simulink model "PMSMWithThermal"  (R2024b)
settings: Solver=VariableStepAuto  StartTime=0.0  StopTime=5  RelTol=1e-3  AbsTol=1e-3
PreLoadFcn:
  | PMSMWithThermalParameters;
values from neighbouring files (symbols this model uses):
  B = 0    [param.mat]
  dt = 0.5e-4    (= 5e-05)    [PMSMWithThermalParameters.m]    (also in param.mat)
  dt_speed_control = 0.001    [PMSMWithThermalParameters.m]    (also in param.mat)
  ESO_w0 = 0    [param.mat]
  J = 0.02    [param.mat]
  max_power = 50e3    (= 50000)    [PMSMWithThermalParameters.m]    (also in param.mat)
  max_torque = 220    [PMSMWithThermalParameters.m]    (also in param.mat)
  N = 6    [PMSMWithThermalParameters.m]    (also in param.mat)
  Rs = 0.013    [PMSMWithThermalParameters.m]    (also in param.mat = 1.3)
undefined symbols (not defined in the file or in its folder): DiscIntNeverNeededParam
libraries: fl_lib x124, nesl_utility x33, fl_ps_legacy_lib x3, ee_lib x1, simulink x1
(part 1 of 2)
CloseFcn:
  | try,close(h1_PMSMWithThermal),end
  | clear h1_PMSMWithThermal
  | try,close(h2_PMSMWithThermal),end
  | clear h2_PMSMWithThermal
  | 
  | 
  | clear simlog_PMSMWithThermal
  | clear logsout_PMSMWithThermal
  | clear Lm Ls Ms N PM Rs dfluxdiMatrix dfluxdxMatrix dt dt_speed_control iVec_th max_power max_torque ni nx row row_PM row_RM tout w_max_power xVecRad xVec_th
Description:
  | PMSM with Thermal Model
settings Model: Creator=The MathWorks, Inc.  LastModifiedBy=Yusuke Seki
settings SolverCC: AutoScaleAbsTol=off  AlgebraicLoopSolver=TrustRegion  MaxZcPerStep=1
settings DataIOCC: MaxDataPoints=210000  SaveFormat=Array  SignalLoggingName=logsout_PMSMWithThermal
settings OptimizationCC: BlockReduction=off  BooleanDataType=off  ReuseModelBlockBuffer=off  LifeSpan=inf
settings DebuggingCC: SaveWithParameterizedLinksMsg=none  SignalResolutionControl=TryResolveAllWithWarning  UnconnectedInputMsg=warning  UnconnectedOutputMsg=warning  UnconnectedLineMsg=warning  AllowSymbolicDim=off  SFUnexpectedBacktrackingDiag=warning  SFNoUnconditionalDefaultTransitionDiag=warning  SFExecutionAtInitializationDiag=none  ArithmeticOperatorsInVariantConditions=warning
settings HardwareCC: ProdBitPerPointer=32  ProdBitPerSizeT=32  ProdBitPerPtrDiffT=32  ProdLargestAtomicFloat=None  ProdIntDivRoundTo=Undefined  ProdEndianess=Unspecified  ProdWordSize=32  ProdHWDeviceType=32-bit Generic  TargetUnknown=on
settings ModelReferenceCC: EnableRefExpFcnMdlSchedulingChecks=on  PropagateSignalLabelsOutOfModel=off
settings SFSimCC: SimUseLocalCustomCode=off  CustomCodeUndefinedFunction=UseInterfaceOnly
settings RTWCC: RTWUseLocalCustomCode=off  GPUComputeCapability=3.5  DLArmComputeVersion=19.05
settings CodeAppCC: StateflowObjectComments=on
settings GRTTargetCC: TargetLangStandard=C89/C90 (ANSI)
settings ConfigComp: CovMetricSettings=dw  CovSaveCumulativeToWorkspaceVar=on  CovSaveSingleToWorkspaceVar=on  CovExternalEMLEnable=off  CovSFcnEnable=off
settings SimscapeCC: SimscapeLogType=all  SimscapeLogSimulationStatistics=on  SimscapeLogName=simlog_PMSMWithThermal  SimscapeLogDecimation=10  SimscapeLogDataHistory=210000

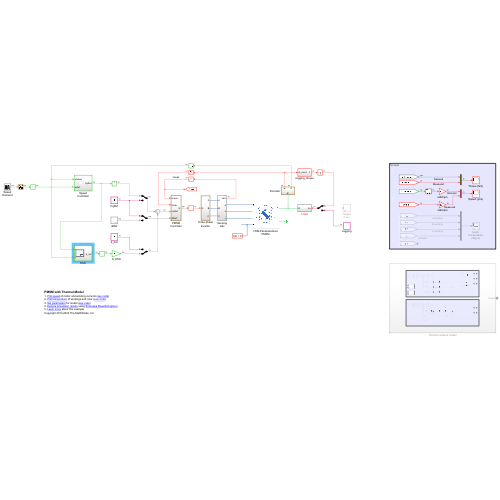
[thumbnail: Simulink's stored preview of the top-level diagram]
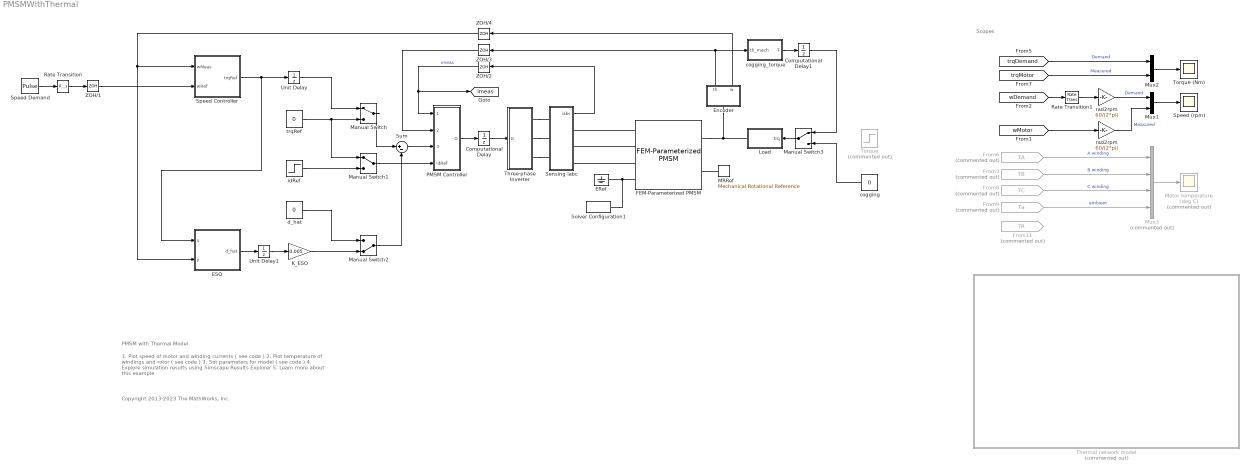
== system PMSMWithThermal ==
  note: Scopes
  note: PMSM with Thermal Model
  note: 1. Plot speed of motor and winding currents ( see code )
      | 2. Plot temperature of windings and rotor ( see code )
      | 3. Set parameters for model ( see code )
      | 4. Explore simulation results using Simscape Results Explorer
      | 5. Learn more about this example
  note: Copyright 2013-2023 The MathWorks, Inc.
  " rad2rpm " : Gain  Gain=60/(2*pi)
  Computational Delay : UnitDelay  SampleTime=dt  HasFrameUpgradeWarning=on
  Computational Delay1 : UnitDelay  SampleTime=dt  HasFrameUpgradeWarning=on
  ERef : fl_lib/Electrical/Electrical Elements/Electrical Reference
  ESO : Subsystem  TreatAsAtomicUnit=on  SystemSampleTime=dt_speed_control
  Encoder : Subsystem
  FEM-Parameterized PMSM : ee_lib/Electromechanical/Permanent Magnet/FEM-Parameterized PMSM  parameterization=ee.enum.fem_motor.parameterization.sinusoidalBackEMF  winding_type=ee.enum.statorconnection.wye  iVec=iVec_th A  xVec=xVec_th deg  dfluxdiMatrix=dfluxdiMatrix Wb/A  dfluxdxMatrix=dfluxdxMatrix Wb/rad  calculate_torque_matrix=1  TorqueMatrix=[0, 0.3, - 0.3, 0; 0, 0, 0, 0; 0, - 0.3, 0.3, 0] N*m  idVec1=[-200.0, 0.0, 200.0] A  iqVec1=[-200.0, 0.0, 200.0] A  LdMatrix=0.0002 * ones(3, 3) H  LqMatrix=0.0002 * ones(3, 3) H  PmMatrix=0.1 * ones(3, 3) Wb  interp_method=1  N=N  Rs=Rs Ohm  Ms=Ms H  L0=0.00016 H  loss_param=ee.enum.fem_motor.ironLosses.none  losses_oc=[0.0, 0.0, 0.0] W  losses_sc=[0.0, 0.0, 0.0] W  f_losses=60 Hz  Isc_losses=95 A  Inertia=J kg*m^2  lam=B N*m/(rad/s)  i_d_specify=off  i_d_priority=None  i_d=0 A  i_d_nominal_specify=off  i_d_nominal_value=1  i_d_nominal_unit=A  i_q_specify=off  i_q_priority=None  i_q=0 A  i_q_nominal_specify=off  i_q_nominal_value=1  i_q_nominal_unit=A  torque_specify=off  torque_priority=None  torque=0 N*m  torque_nominal_specify=off  torque_nominal_value=1  torque_nominal_unit=N*m  angular_velocity_specify=on  angular_velocity_priority=High  angular_velocity=0 rpm  angular_velocity_nominal_specify=off  angular_velocity_nominal_value=1  angular_velocity_nominal_unit=rpm  angular_position_specify=on  angular_position_priority=High  angular_position=0 deg  angular_position_nominal_specify=off  angular_position_nominal_value=1  angular_position_nominal_unit=deg  alpha=3.93e-3 1/K  alpha_flux=-0.001 1/K  Tmeas=298.15 K  stator_thermal_mass=2 J/K  stator_initial_temperatures=[298.15, 298.15, 298.15] K  rotor_thermal_mass=20 J/K  rotor_initial_temperature=298.15 K  Rm_percent_rotor=90  Rd_percent_rotor=30  idVec=[-200, 0, 200] A  iqVec=[-200, 0, 200] A  dfluxAdiaMatrix3D=zeros(3, 3, 4) Wb/A  dfluxAdibMatrix3D=zeros(3, 3, 4) Wb/A  dfluxAdicMatrix3D=zeros(3, 3, 4) Wb/A  dfluxAdxMatrix3D=zeros(3, 3, 4) Wb/rad  TorqueMatrix3D=zeros(3, 3, 4) N*m  iaVec=[-200, 0, 200] A  ibVec=[-200, 0, 200] A  icVec=[-200, 0, 200] A  dfluxAdiaMatrix=zeros(3, 3, 3, 4) Wb/A  dfluxAdibMatrix=zeros(3, 3, 3, 4) Wb/A  dfluxAdicMatrix=zeros(3, 3, 3, 4) Wb/A  dfluxAdxMatrix=zeros(3, 3, 3, 4) Wb/rad  param_dq0=ee.enum.fem_motor.fluxTabulationOption.DQcartesian  winding_type_dq0=ee.enum.statorconnection.wye  expose_neutral_port=ee.enum.fem_motor.exposeNeutralPort.no  nPolePairs=4  parks_type=ee.enum.fem_motor.parksType.QleadsD_AphaseToDaxis  idVec2=[-200, 0, 200] A  iqVec2=[-200, 0, 200] A  magVec2=[0, 100, 200] A  betaVec2=[-180, -90, 0, 90, 180] deg  xVec2=[0, 5, 10, 15, 20, 25, 30] deg  fluxD_dq0=zeros(3, 3, 7) Wb  fluxQ_dq0=zeros(3, 3, 7) Wb  fluxA_dq0=zeros(3, 3, 7) Wb  Torque_dq0=ones(3, 3, 7) N*m  fluxD_IBX=zeros(3, 5, 7) Wb  fluxQ_IBX=zeros(3, 5, 7) Wb  fluxA_IBX=zeros(3, 5, 7) Wb  Torque_IBX=zeros(3, 5, 7) N*m  rotorLossCoeff_k_h_DQ=zeros(3, 3) W/Hz  rotorLossCoeff_k_J_DQ=zeros(3, 3) W/Hz^2  rotorLossCoeff_k_ex_DQ=zeros(3, 3) W/Hz^(3/2)  rotorLossCoeff_k_h_IB=zeros(3, 5) W/Hz  rotorLossCoeff_k_J_IB=zeros(3, 5) W/Hz^2  rotorLossCoeff_k_ex_IB=zeros(3, 5) W/Hz^(3/2)  statorLossCoeff_k_h_DQ=zeros(3, 3) W/Hz  statorLossCoeff_k_J_DQ=zeros(3, 3) W/Hz^2  statorLossCoeff_k_ex_DQ=zeros(3, 3) W/Hz^(3/2)  statorLossCoeff_k_h_IB=zeros(3, 5) W/Hz  statorLossCoeff_k_J_IB=zeros(3, 5) W/Hz^2  statorLossCoeff_k_ex_IB=zeros(3, 5) W/Hz^(3/2)  wVec=[1000, 2000] rpm  rotorLossTable_DQ=zeros(3, 3, 2) W  statorLossTable_DQ=zeros(3, 3, 2) W  rotorLossTable_IB=zeros(3, 5, 2) W  statorLossTable_IB=zeros(3, 5, 2) W  electrical_torque_before_iron_losses_specify=off  electrical_torque_before_iron_losses_priority=None  electrical_torque_before_iron_losses=0 N*m  electrical_torque_before_iron_losses_nominal_specify=off  electrical_torque_before_iron_losses_nominal_value=1  electrical_torque_before_iron_losses_nominal_unit=N*m  Qrotor_specify=off  Qrotor_priority=None  Qrotor=0 J/s  Qrotor_nominal_specify=off  Qrotor_nominal_value=1  Qrotor_nominal_unit=J/s  Qstator_specify=off  Qstator_priority=None  Qstator=0 J/s  Qstator_nominal_specify=off  Qstator_nominal_value=1  Qstator_nominal_unit=J/s
      settings: InternalSimscapePortConfiguration="{\"Bottom\":[],\"Left\":[{\"id\":\"a\",\"label\":\"a\",\"type\":\"foundation.electrical.electrical\"},{\"id\":\"b\",\"label\":\"b\",\"type\":\"foundation.electrical.electrical\"},{\"id\":\"c\",\"label\":\"c\",\"type\":\"foundation.electrical.electrical\"},{\"id\":\"n\",\"label\":\"n\",\"type\":\"foundation.electrical.electrical\"}],\"Right\":[{\"id\":\"R\",\"label\":\"R\",\"type\":\"foundation.mechanical.rotational.rotational\"},{\"id\":\"C\",\"label\":\"C\",\"type\":\"foundation.mechanical.rotational.rotational\"}],\"Top\":[]}"
  From11 : From  Commented=on  GotoTag=TR  TagVisibility=global
  From3 : From  Commented=on  GotoTag=TB  TagVisibility=global
  From6 : From  Commented=on  GotoTag=TA  TagVisibility=global
  From8 : From  Commented=on  GotoTag=TC  TagVisibility=global
  From9 : From  Commented=on  GotoTag=Ta  TagVisibility=global
  K_ESO : Gain  Gain=0.005
  Load : Subsystem
  MRRef : fl_lib/Mechanical/Rotational Elements/Mechanical Rotational Reference
  Manual Switch : ManualSwitch
  Manual Switch1 : ManualSwitch
  Manual Switch2 : ManualSwitch  CurrentSetting=0
  Manual Switch3 : ManualSwitch
  Motor temperature (deg C) : Scope  Commented=on
  Mux1 : Mux  Inputs=2
  Mux2 : Mux  Inputs=2
  Mux3 : Mux  Commented=on
  PMSM Controller : Subsystem
  Rate Transition : RateTransition
  Rate Transition1 : RateTransition
  Sensing iabc : Subsystem
  Solver Configuration1 : nesl_utility/Solver Configuration  PhysicalDomain=network_engine_domain  SubClassName=solver  LeftPortType=input  RightPortType=generic  Tones=[]  Harmonics=[]  SimulateNoise=off  Profile=off  UseLocalSampling=off  EnableSwitchedLinearOptims=on  FrequencyDomain=off  UseCCode=off  RelTol=0.001  AbsTol=1e-06  MinStep=1e-09  ToWorkspace=off  RevertToSquareIcSolve=off  NumHomotopyIterations=100  PhasorMode=off  PhasorModeNumHarmonics=1  ConsistencySolver=NEWTON_XTOL_AFTER_FTOL  IndexReductionMethod=DerivativeReplacement  DoDC=off  ResidualTolerance=1e-9  ConsistencyTolSource=GLOBAL  ConsistencyAbsTol=0.001  ConsistencyRelTol=0.001  ConsistencyTolFactor=0.001  UseLocalSolver=on  LocalSolverChoice=NE_BACKWARD_EULER_ADVANCER  ResolveIndetEquations=on  FunctionEvalNumThread=1  LocalSolverSampleTime=dt  DoFixedCost=on  MaxNonlinIter=3  MaxModeIter=2  ComputeImpulses=off  ImpulseIterations=2  LinearAlgebra=auto  LinearAlgebraNumThread=0  EquationFormulation=NE_TIME_EF  DelaysMemoryBudget=1024  AutomaticFiltering=on  FilteringTimeConstant=0.001  PartitionStorageMethod=AS_NEEDED  PartitionMemoryBudget=1024  PartitionMethod=FAST  MultibodyUseLocalSolver=off  MultibodyLocalSolverChoice=ODE1  MultibodyLocalSolverSampleTime=0.001
  Speed Controller : Subsystem  SystemSampleTime=dt_speed_control
  Speed Demand : DiscretePulseGenerator  PulseType=Time based  Amplitude=200*2*pi/60  Period=10  PulseWidth=30  PhaseDelay=0.2
  Speed (rpm) : Scope
  Sum : Sum  Inputs=|+-
  Thermal network model : Subsystem  Commented=on
  Three-phase Inverter : Subsystem  VariantControl=Variant
  Torque : Step  Commented=on  Time=5  After=0  SampleTime=dt
      settings: AttributesFormatString=%<Time> sec
  Torque (Nm) : Scope
  Unit Delay : UnitDelay  SampleTime=dt_speed_control  HasFrameUpgradeWarning=on
  Unit Delay1 : UnitDelay  SampleTime=dt_speed_control  HasFrameUpgradeWarning=on
  ZOH/1 : ZeroOrderHold  SampleTime=dt_speed_control
  ZOH/2 : ZeroOrderHold  SampleTime=dt
  ZOH/3 : ZeroOrderHold  SampleTime=dt
  ZOH/4 : ZeroOrderHold  SampleTime=dt_speed_control
  cogging : Constant  Value=0
  cogging_torque : Subsystem
  d_hat : Constant  Value=0
  idRef : Step  Time=50  Before=10  After=0  SampleTime=0
  rad2rpm : Gain  Gain=60/(2*pi)
  trqRef : Constant  Value=0
  tag scope: imeas=global
  wires:
  Encoder/2(w) -> ZOH/4/1
  Speed Demand/1 -> Rate Transition/1
  ZOH/1/1 -> Speed Controller/2(wRef)
  ZOH/3/1 -> PMSM Controller/2(theta)
  ZOH/2/1 -> [imeas], PMSM Controller/1(imeas)  "imeas"
  PMSM Controller/1(G) -> Computational Delay/1
  Encoder/1(th) -> cogging_torque/1(th_mech), ZOH/3/1
  Computational Delay/1 -> Three-phase Inverter/1(G)
  Sensing iabc/1(iabc) -> ZOH/2/1
  Rate Transition/1 -> ZOH/1/1
  Unit Delay/1 -> Manual Switch/1
  From8/1 -> Mux3/3  "C winding"
  Mux3/1 -> Motor temperature (deg C)/1
  From6/1 -> Mux3/1  "A winding"
  [trqMotor] -> Mux2/2  "Measured"
  [trqDemand] -> Mux2/1  "Demand"
  Rate Transition1/1 -> rad2rpm/1
  Mux2/1 -> Torque (Nm)/1
  [wMotor] -> " rad2rpm "/1
  " rad2rpm "/1 -> Mux1/2  "Measured"
  [wDemand] -> Rate Transition1/1
  From3/1 -> Mux3/2  "B winding"
  rad2rpm/1 -> Mux1/1  "Demand"
  Mux1/1 -> Speed (rpm)/1
  From9/1 -> Mux3/4  "ambient"
  trqRef/1 -> Manual Switch1/1, Manual Switch/2
  Manual Switch1/1 -> PMSM Controller/4(idRef)
  idRef/1 -> Manual Switch1/2
  cogging_torque/1(T) -> Computational Delay1/1
  Computational Delay1/1 -> Manual Switch3/1
  ZOH/4/1 -> ESO/2(y), Speed Controller/1(wMeas)
  Manual Switch/1 -> Sum/1
  Sum/1 -> PMSM Controller/3(trqRef)
  d_hat/1 -> Manual Switch2/1
  Manual Switch2/1 -> Sum/2
  Manual Switch3/1 -> Load/1(trq)
  cogging/1 -> Manual Switch3/2
  Speed Controller/1(trqRef) -> Unit Delay/1, ESO/1(u)
  K_ESO/1 -> Manual Switch2/2
  ESO/1(d_hat) -> Unit Delay1/1
  Unit Delay1/1 -> K_ESO/1
  connections:
  Solver Configuration1/RConn1 -- FEM-Parameterized PMSM/LConn4 -- ERef/LConn1
  MRRef/LConn1 -- FEM-Parameterized PMSM/RConn2
  FEM-Parameterized PMSM/RConn1 -- Load/RConn1 -- Encoder/LConn1
  Three-phase Inverter/RConn1 -- Sensing iabc/LConn1
  FEM-Parameterized PMSM/LConn1 -- Sensing iabc/RConn1
  Three-phase Inverter/RConn2 -- Sensing iabc/LConn2
  FEM-Parameterized PMSM/LConn2 -- Sensing iabc/RConn2
  Three-phase Inverter/RConn3 -- Sensing iabc/LConn3
  FEM-Parameterized PMSM/LConn3 -- Sensing iabc/RConn3

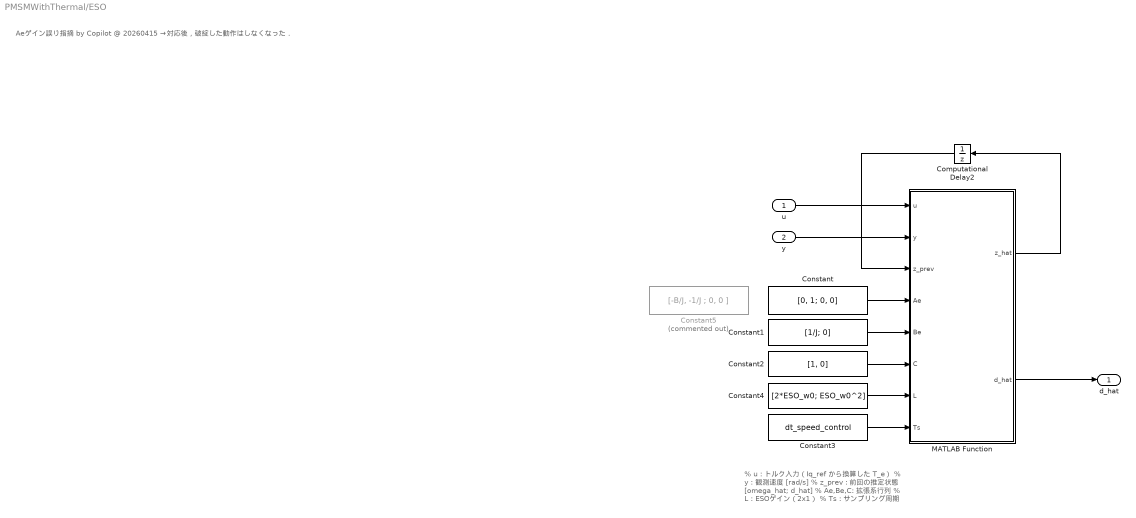
== system PMSMWithThermal/ESO ==
  note: Aeゲイン誤り指摘 by Copilot @ 20260415
      | →対応後，破綻した動作はしなくなった．
  note: % u : トルク入力（Iq_ref から換算した T_e）
      | % y : 観測速度 [rad/s]
      | % z_prev : 前回の推定状態 [omega_hat; d_hat]
      | % Ae,Be,C: 拡張系行列
      | % L : ESOゲイン（2x1）
      | % Ts : サンプリング周期
  u : Inport
  y : Inport  Port=2
  Computational Delay2 : UnitDelay  InitialCondition=[0; 0]  SampleTime=dt_speed_control  HasFrameUpgradeWarning=on
  Constant : Constant  Value=[0, 1; 0, 0]  VectorParams1D=off
  Constant1 : Constant  Value=[1/J; 0]  VectorParams1D=off
  Constant2 : Constant  Value=[1, 0]  VectorParams1D=off
  Constant3 : Constant  Value=dt_speed_control  VectorParams1D=off
  Constant4 : Constant  Value=[2*ESO_w0; ESO_w0^2]  VectorParams1D=off
  Constant5 : Constant  Commented=on  Value=[-B/J, -1/J ; 0, 0 ]  VectorParams1D=off
  MATLAB Function : MATLAB Function  TreatAsAtomicUnit=on  SystemSampleTime=dt_speed_control
  d_hat : Outport
  wires:
  Constant1/1 -> MATLAB Function/5(Be)
  Constant/1 -> MATLAB Function/4(Ae)
  Constant3/1 -> MATLAB Function/8(Ts)
  Constant4/1 -> MATLAB Function/7(L)
  Constant2/1 -> MATLAB Function/6(C)
  y/1 -> MATLAB Function/2(y)
  u/1 -> MATLAB Function/1(u)
  MATLAB Function/1(z_hat) -> Computational Delay2/1
  MATLAB Function/2(d_hat) -> d_hat/1
  Computational Delay2/1 -> MATLAB Function/3(z_prev)

== system PMSMWithThermal/Encoder ==
  MRRef : fl_lib/Mechanical/Rotational Elements/Mechanical Rotational Reference
  Motion Sensor : fl_lib/Mechanical/Mechanical Sensors/Ideal Rotational Motion Sensor  reference=foundation.enum.MeasurementReference.difference  acceleration_port=false  velocity_port=true  position_port=true  wrap_angle=true  offset=0 rad
  PS-Simulink Converter : nesl_utility/PS-Simulink Converter  PhysicalDomain=network_engine_domain  SubClassName=ps_output  LeftPortType=input  RightPortType=output  PseudoPeriodic=off  Frequencies=[]  VectorFormat=1-D array  Unit=rad/s  AffineConversion=off
  PS-Simulink Converter1 : nesl_utility/PS-Simulink Converter  PhysicalDomain=network_engine_domain  SubClassName=ps_output  LeftPortType=input  RightPortType=output  PseudoPeriodic=off  Frequencies=[]  VectorFormat=1-D array  Unit=rad  AffineConversion=off
  Rate Transition : RateTransition
  R : PMIOPort  Side=Left
  th : Outport  VectorParamsAs1DForOutWhenUnconnected=off
  w : Outport  Port=2  VectorParamsAs1DForOutWhenUnconnected=off
  tag scope: wMotor=global
  wires:
  PS-Simulink Converter/1 -> [wMotor], Rate Transition/1
  PS-Simulink Converter1/1 -> th/1
  Rate Transition/1 -> w/1
  connections:
  MRRef/LConn1 -- Motion Sensor/RConn1
  Motion Sensor/LConn1 -- R/RConn1
  PS-Simulink Converter1/LConn1 -- Motion Sensor/RConn3
  PS-Simulink Converter/LConn1 -- Motion Sensor/RConn2

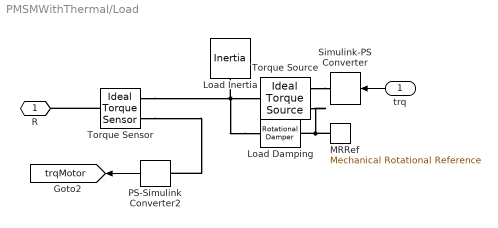
== system PMSMWithThermal/Load ==
  trq : Inport
  Load Damping : fl_lib/Mechanical/Rotational Elements/Rotational Damper  D=30e3/(2*pi/60*2000)^2 N*m/(rad/s)  w_specify=off  w_priority=None  w=0 rad/s  w_nominal_specify=off  w_nominal_value=1  w_nominal_unit=rad/s  t_specify=off  t_priority=None  t=0 N*m  t_nominal_specify=off  t_nominal_value=1  t_nominal_unit=N*m
  Load Inertia : fl_lib/Mechanical/Rotational Elements/Inertia  inertia=1 kg*m^2  num_ports=foundation.enum.numPorts2.one  w_specify=off  w_priority=None  w=0 rad/s  w_nominal_specify=off  w_nominal_value=1  w_nominal_unit=rad/s  t_specify=off  t_priority=None  t=0 N*m  t_nominal_specify=off  t_nominal_value=1  t_nominal_unit=N*m
  MRRef : fl_lib/Mechanical/Rotational Elements/Mechanical Rotational Reference
  PS-Simulink Converter2 : nesl_utility/PS-Simulink Converter  PhysicalDomain=network_engine_domain  SubClassName=ps_output  LeftPortType=input  RightPortType=output  PseudoPeriodic=off  Frequencies=[]  VectorFormat=1-D array  Unit=N*m  AffineConversion=off
  Simulink-PS Converter : nesl_utility/Simulink-PS Converter  PhysicalDomain=network_engine_domain  SubClassName=ps_input  LeftPortType=input  RightPortType=output  PseudoPeriodic=off  Frequencies=[]  NoiseDistribution=none  NoiseParameters=[]  Unit=1  AffineConversion=off  FilteringAndDerivatives=zero  SimscapeFilterOrder=1  InputFilterTimeConstant=0.001  UdotUserProvided=1
  Torque Source : fl_lib/Mechanical/Mechanical Sources/Ideal Torque Source
  Torque Sensor : fl_lib/Mechanical/Mechanical Sensors/Ideal Torque Sensor
  R : PMIOPort  Side=Right
  tag scope: trqMotor=global
  wires:
  trq/1 -> Simulink-PS Converter/1
  PS-Simulink Converter2/1 -> [trqMotor]
  connections:
  Torque Source/RConn1 -- Simulink-PS Converter/RConn1
  MRRef/LConn1 -- Torque Source/RConn2 -- Load Damping/RConn1
  Load Damping/LConn1 -- Torque Sensor/RConn1 -- Load Inertia/LConn1 -- Torque Source/LConn1
  Torque Sensor/LConn1 -- R/RConn1
  Torque Sensor/RConn2 -- PS-Simulink Converter2/LConn1

== system PMSMWithThermal/PMSM Controller ==
  imeas : Inport
  theta : Inport  Port=2
  trqRef : Inport  Port=3
  idRef : Inport  Port=4
  Rate Transition : RateTransition
  Vector controller : Subsystem  mask(Vector controller){Np=6, lambda=0.1, h=10}
      mask prompts: Np "Number of pole pairs, p"; lambda "Flux linkage from rotor permanent magnet"; h "Current hysteresis (A)"
  G : Outport  VectorParamsAs1DForOutWhenUnconnected=off
  tag scope: trqDemand=global
  wires:
  theta/1 -> Vector controller/2(theta)
  imeas/1 -> Vector controller/3(I_abc)
  trqRef/1 -> Rate Transition/1
  Vector controller/1(G) -> G/1
  Rate Transition/1 -> [trqDemand], Vector controller/1(trqRef)
  idRef/1 -> Vector controller/4(idRef)

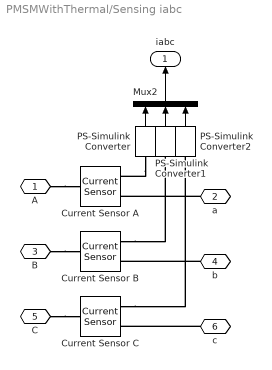
== system PMSMWithThermal/Sensing iabc ==
  Current Sensor A : fl_lib/Electrical/Electrical Sensors/Current Sensor
  Current Sensor B : fl_lib/Electrical/Electrical Sensors/Current Sensor
  Current Sensor C : fl_lib/Electrical/Electrical Sensors/Current Sensor
  Mux2 : Mux  Inputs=[1,1,1]
  PS-Simulink Converter : nesl_utility/PS-Simulink Converter  PhysicalDomain=network_engine_domain  SubClassName=ps_output  LeftPortType=input  RightPortType=output  PseudoPeriodic=off  Frequencies=[]  VectorFormat=1-D array  Unit=A  AffineConversion=off
  PS-Simulink Converter1 : nesl_utility/PS-Simulink Converter  PhysicalDomain=network_engine_domain  SubClassName=ps_output  LeftPortType=input  RightPortType=output  PseudoPeriodic=off  Frequencies=[]  VectorFormat=1-D array  Unit=A  AffineConversion=off
  PS-Simulink Converter2 : nesl_utility/PS-Simulink Converter  PhysicalDomain=network_engine_domain  SubClassName=ps_output  LeftPortType=input  RightPortType=output  PseudoPeriodic=off  Frequencies=[]  VectorFormat=1-D array  Unit=A  AffineConversion=off
  A : PMIOPort  Side=Left
  a : PMIOPort  Port=2  Side=Right
  B : PMIOPort  Port=3  Side=Left
  b : PMIOPort  Port=4  Side=Right
  C : PMIOPort  Port=5  Side=Left
  c : PMIOPort  Port=6  Side=Right
  iabc : Outport  VectorParamsAs1DForOutWhenUnconnected=off
  wires:
  PS-Simulink Converter/1 -> Mux2/1
  PS-Simulink Converter1/1 -> Mux2/2
  PS-Simulink Converter2/1 -> Mux2/3
  Mux2/1 -> iabc/1
  connections:
  b/RConn1 -- Current Sensor B/RConn2
  A/RConn1 -- Current Sensor A/LConn1
  c/RConn1 -- Current Sensor C/RConn2
  Current Sensor B/RConn1 -- PS-Simulink Converter1/LConn1
  Current Sensor C/RConn1 -- PS-Simulink Converter2/LConn1
  a/RConn1 -- Current Sensor A/RConn2
  C/RConn1 -- Current Sensor C/LConn1
  PS-Simulink Converter/LConn1 -- Current Sensor A/RConn1
  B/RConn1 -- Current Sensor B/LConn1

== system PMSMWithThermal/Speed Controller ==
  wMeas : Inport
  wRef : Inport  Port=2
  Power and torque limits : Subsystem
  Speed controller : Subsystem
  trqRef : Outport  VectorParamsAs1DForOutWhenUnconnected=off
  wires:
  Speed controller/1(trqRef) -> Power and torque limits/2(trqRef)
  wRef/1 -> Speed controller/2(wRef)
  wMeas/1 -> Power and torque limits/1(wMeas), Speed controller/1(wMeas)
  Power and torque limits/1(trqRefLim) -> trqRef/1

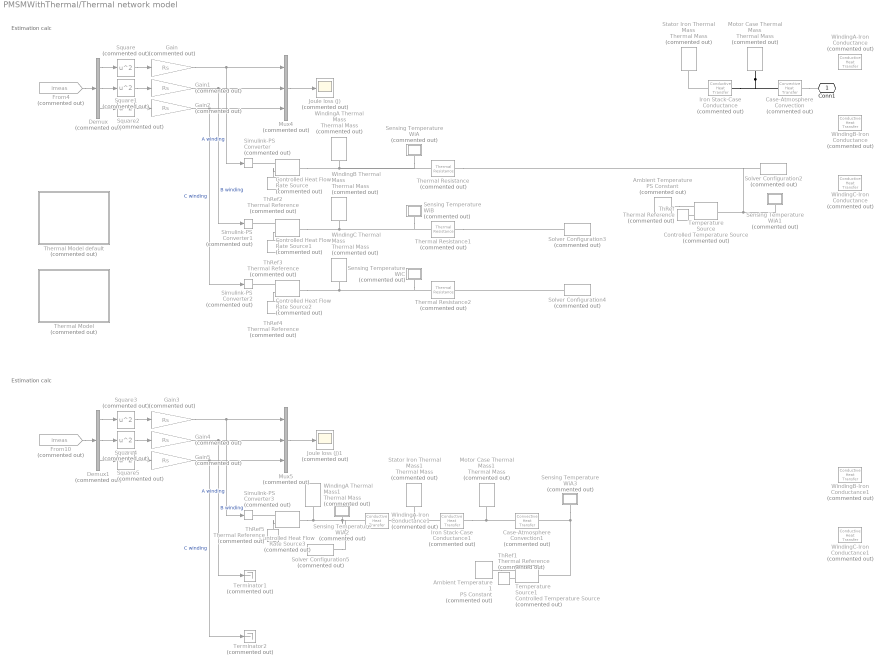
== system PMSMWithThermal/Thermal network model ==
  note: Estimation calc
  note: Estimation calc
  Ambient Temperature : fl_lib/Physical Signals/Sources/PS Constant  Commented=on  constant=300
  Ambient Temperature1 : fl_lib/Physical Signals/Sources/PS Constant  Commented=on  constant=300
  Case-Atmosphere Convection : fl_lib/Thermal/Thermal Elements/Convective Heat Transfer  Commented=on  thermal_type=foundation.enum.constant_variable.constant  area=4240 cm^2  heat_tr_coeff=26.8 W/(m^2 * K)  min_heat_tr_coeff=1e-3 W/(K*m^2)  T_specify=off  T_priority=None  T=0 K  T_nominal_specify=off  T_nominal_value=1  T_nominal_unit=K  Q_specify=off  Q_priority=None  Q=0 W  Q_nominal_specify=off  Q_nominal_value=1  Q_nominal_unit=W
  Case-Atmosphere Convection1 : fl_lib/Thermal/Thermal Elements/Convective Heat Transfer  Commented=on  thermal_type=foundation.enum.constant_variable.constant  area=4240 cm^2  heat_tr_coeff=26.8 W/(m^2 * K)  min_heat_tr_coeff=1e-3 W/(K*m^2)  T_specify=off  T_priority=None  T=0 K  T_nominal_specify=off  T_nominal_value=1  T_nominal_unit=K  Q_specify=off  Q_priority=None  Q=0 W  Q_nominal_specify=off  Q_nominal_value=1  Q_nominal_unit=W
  Controlled Heat Flow Rate Source{,1..3} (4 alike) : fl_lib/Thermal/Thermal Sources/Controlled Heat Flow Rate Source  Commented=on
  Demux : Demux  Commented=on  Outputs=3
  Demux1 : Demux  Commented=on  Outputs=3
  From10 : From  Commented=on  GotoTag=imeas  TagVisibility=global
  From4 : From  Commented=on  GotoTag=imeas  TagVisibility=global
  Gain{,1..5} (6 alike) : Gain  Commented=on  Gain=Rs
  Iron Stack-Case Conductance : fl_lib/Thermal/Thermal Elements/Conductive Heat Transfer  Commented=on  thermal_type=foundation.enum.ConstantVariableTabulated.Constant  wall_geometry=foundation.enum.ConductionWallGeometry.Planar  area=4350 cm^2  thickness=26 cm  d_in=0.05 m  d_out=0.1 m  L=1 m  th_cond_min=10 W/(K*m)  th_cond=80.2 W/(m*K)  th_cond_TLU=[413, 401, 392, 383, 371, 357, 342] W/(K*m)  temp_TLU=[200, 273, 400, 600, 800, 1000, 1200] K  T_specify=off  T_priority=None  T=0 K  T_nominal_specify=off  T_nominal_value=1  T_nominal_unit=K  Q_specify=off  Q_priority=None  Q=0 W  Q_nominal_specify=off  Q_nominal_value=1  Q_nominal_unit=W
  Iron Stack-Case Conductance1 : fl_lib/Thermal/Thermal Elements/Conductive Heat Transfer  Commented=on  thermal_type=foundation.enum.ConstantVariableTabulated.Constant  wall_geometry=foundation.enum.ConductionWallGeometry.Planar  area=4350 cm^2  thickness=26 cm  d_in=0.05 m  d_out=0.1 m  L=1 m  th_cond_min=10 W/(K*m)  th_cond=80.2 W/(m*K)  th_cond_TLU=[413, 401, 392, 383, 371, 357, 342] W/(K*m)  temp_TLU=[200, 273, 400, 600, 800, 1000, 1200] K  T_specify=off  T_priority=None  T=0 K  T_nominal_specify=off  T_nominal_value=1  T_nominal_unit=K  Q_specify=off  Q_priority=None  Q=0 W  Q_nominal_specify=off  Q_nominal_value=1  Q_nominal_unit=W
  Joule loss (J) : Scope  Commented=on
  Joule loss (J)1 : Scope  Commented=on
  Motor Case Thermal Mass : fl_lib/Thermal/Thermal Elements/Thermal Mass  Commented=on  mass_type=foundation.enum.constant_variable.constant  mass=3.8 kg  sp_heat=903 J/kg/K  mass_min=1e-6 kg  num_ports=foundation.enum.numPorts2.one  m_specify=off  m_priority=High  m=1 kg  m_nominal_specify=off  m_nominal_value=1  m_nominal_unit=kg  T_specify=off  T_priority=High  T=300 K  T_nominal_specify=off  T_nominal_value=1  T_nominal_unit=K  Q_specify=off  Q_priority=None  Q=0 W  Q_nominal_specify=off  Q_nominal_value=1  Q_nominal_unit=W
  Motor Case Thermal Mass1 : fl_lib/Thermal/Thermal Elements/Thermal Mass  Commented=on  mass_type=foundation.enum.constant_variable.constant  mass=3.8 kg  sp_heat=903 J/kg/K  mass_min=1e-6 kg  num_ports=foundation.enum.numPorts2.one  m_specify=off  m_priority=High  m=1 kg  m_nominal_specify=off  m_nominal_value=1  m_nominal_unit=kg  T_specify=off  T_priority=High  T=300 K  T_nominal_specify=off  T_nominal_value=1  T_nominal_unit=K  Q_specify=off  Q_priority=None  Q=0 W  Q_nominal_specify=off  Q_nominal_value=1  Q_nominal_unit=W
  Mux4 : Mux  Commented=on  Inputs=3
  Mux5 : Mux  Commented=on  Inputs=3
  Sensing Temperature WiA : Subsystem  Commented=on
      mask Display: disp('TA')
  Sensing Temperature WiA1 : Subsystem  Commented=on
      mask Display: disp('TA')
  Sensing Temperature WiA2 : Subsystem  Commented=on
      mask Display: disp('TA')
  Sensing Temperature WiA3 : Subsystem  Commented=on
      mask Display: disp('TA')
  Sensing Temperature WiB : Subsystem  Commented=on
      mask Display: disp('TB')
  Sensing Temperature WiC : Subsystem  Commented=on
      mask Display: disp('TC')
  Simulink-PS Converter{,1..3} (4 alike) : nesl_utility/Simulink-PS Converter  Commented=on  PhysicalDomain=network_engine_domain  SubClassName=ps_input  LeftPortType=input  RightPortType=output  PseudoPeriodic=off  Frequencies=[]  NoiseDistribution=none  NoiseParameters=[]  Unit=J/s  AffineConversion=off  FilteringAndDerivatives=provide  SimscapeFilterOrder=1  InputFilterTimeConstant=0.001  UdotUserProvided=0
  Solver Configuration{2..5} (4 alike) : nesl_utility/Solver Configuration  Commented=on  PhysicalDomain=network_engine_domain  SubClassName=solver  LeftPortType=input  RightPortType=generic  Tones=[]  Harmonics=[]  SimulateNoise=off  Profile=off  UseLocalSampling=off  EnableSwitchedLinearOptims=on  FrequencyDomain=off  UseCCode=off  RelTol=0.001  AbsTol=1e-06  MinStep=1e-09  ToWorkspace=off  RevertToSquareIcSolve=off  NumHomotopyIterations=100  PhasorMode=off  PhasorModeNumHarmonics=1  ConsistencySolver=NEWTON_XTOL_AFTER_FTOL  IndexReductionMethod=DerivativeReplacement  DoDC=off  ResidualTolerance=1e-9  ConsistencyTolSource=GLOBAL  ConsistencyAbsTol=0.001  ConsistencyRelTol=0.001  ConsistencyTolFactor=0.001  UseLocalSolver=on  LocalSolverChoice=NE_BACKWARD_EULER_ADVANCER  ResolveIndetEquations=on  FunctionEvalNumThread=1  LocalSolverSampleTime=dt  DoFixedCost=on  MaxNonlinIter=3  MaxModeIter=2  ComputeImpulses=off  ImpulseIterations=2  LinearAlgebra=auto  LinearAlgebraNumThread=0  EquationFormulation=NE_TIME_EF  DelaysMemoryBudget=1024  AutomaticFiltering=on  FilteringTimeConstant=0.001  PartitionStorageMethod=AS_NEEDED  PartitionMemoryBudget=1024  PartitionMethod=FAST  MultibodyUseLocalSolver=off  MultibodyLocalSolverChoice=ODE1  MultibodyLocalSolverSampleTime=0.001
  Square{,1..5} (6 alike) : Math  Commented=on  Operator=square
  Stator Iron Thermal Mass : fl_lib/Thermal/Thermal Elements/Thermal Mass  Commented=on  mass_type=foundation.enum.constant_variable.constant  mass=4.1 kg  sp_heat=447 J/kg/K  mass_min=1e-6 kg  num_ports=foundation.enum.numPorts2.one  m_specify=off  m_priority=High  m=1 kg  m_nominal_specify=off  m_nominal_value=1  m_nominal_unit=kg  T_specify=off  T_priority=High  T=300 K  T_nominal_specify=off  T_nominal_value=1  T_nominal_unit=K  Q_specify=off  Q_priority=None  Q=0 W  Q_nominal_specify=off  Q_nominal_value=1  Q_nominal_unit=W
  Stator Iron Thermal Mass1 : fl_lib/Thermal/Thermal Elements/Thermal Mass  Commented=on  mass_type=foundation.enum.constant_variable.constant  mass=4.1 kg  sp_heat=447 J/kg/K  mass_min=1e-6 kg  num_ports=foundation.enum.numPorts2.one  m_specify=off  m_priority=High  m=1 kg  m_nominal_specify=off  m_nominal_value=1  m_nominal_unit=kg  T_specify=off  T_priority=High  T=300 K  T_nominal_specify=off  T_nominal_value=1  T_nominal_unit=K  Q_specify=off  Q_priority=None  Q=0 W  Q_nominal_specify=off  Q_nominal_value=1  Q_nominal_unit=W
  Temperature Source : fl_lib/Thermal/Thermal Sources/Controlled Temperature Source  Commented=on
  Temperature Source1 : fl_lib/Thermal/Thermal Sources/Controlled Temperature Source  Commented=on
  Terminator1 : Terminator  Commented=on
  Terminator2 : Terminator  Commented=on
  ThRef{,1..5} (6 alike) : fl_lib/Thermal/Thermal Elements/Thermal Reference  Commented=on
  Thermal Model : Subsystem  Tag=PublishSubsystem  Commented=on
  Thermal Model default : Subsystem  Tag=PublishSubsystem  Commented=on
  Thermal Resistance : fl_lib/Thermal/Thermal Elements/Thermal Resistance  Commented=on  resistance=1 K/W  T_specify=off  T_priority=None  T=0 K  T_nominal_specify=off  T_nominal_value=1  T_nominal_unit=K  Q_specify=off  Q_priority=None  Q=0 W  Q_nominal_specify=off  Q_nominal_value=1  Q_nominal_unit=W
  Thermal Resistance1 : fl_lib/Thermal/Thermal Elements/Thermal Resistance  Commented=on  resistance=1 K/W  T_specify=off  T_priority=None  T=0 K  T_nominal_specify=off  T_nominal_value=1  T_nominal_unit=K  Q_specify=off  Q_priority=None  Q=0 W  Q_nominal_specify=off  Q_nominal_value=1  Q_nominal_unit=W
  Thermal Resistance2 : fl_lib/Thermal/Thermal Elements/Thermal Resistance  Commented=on  resistance=1 K/W  T_specify=off  T_priority=None  T=0 K  T_nominal_specify=off  T_nominal_value=1  T_nominal_unit=K  Q_specify=off  Q_priority=None  Q=0 W  Q_nominal_specify=off  Q_nominal_value=1  Q_nominal_unit=W
  WindingA Thermal Mass : fl_lib/Thermal/Thermal Elements/Thermal Mass  Commented=on  mass_type=foundation.enum.constant_variable.constant  mass=6.3 kg  sp_heat=385 J/kg/K  mass_min=1e-6 kg  num_ports=foundation.enum.numPorts2.one  m_specify=off  m_priority=High  m=1 kg  m_nominal_specify=off  m_nominal_value=1  m_nominal_unit=kg  T_specify=off  T_priority=High  T=300 K  T_nominal_specify=off  T_nominal_value=1  T_nominal_unit=K  Q_specify=off  Q_priority=None  Q=0 W  Q_nominal_specify=off  Q_nominal_value=1  Q_nominal_unit=W
  WindingA Thermal Mass1 : fl_lib/Thermal/Thermal Elements/Thermal Mass  Commented=on  mass_type=foundation.enum.constant_variable.constant  mass=6.3 kg  sp_heat=385 J/kg/K  mass_min=1e-6 kg  num_ports=foundation.enum.numPorts2.one  m_specify=off  m_priority=High  m=1 kg  m_nominal_specify=off  m_nominal_value=1  m_nominal_unit=kg  T_specify=off  T_priority=High  T=300 K  T_nominal_specify=off  T_nominal_value=1  T_nominal_unit=K  Q_specify=off  Q_priority=None  Q=0 W  Q_nominal_specify=off  Q_nominal_value=1  Q_nominal_unit=W
  WindingA-Iron Conductance : fl_lib/Thermal/Thermal Elements/Conductive Heat Transfer  Commented=on  thermal_type=foundation.enum.ConstantVariableTabulated.Constant  wall_geometry=foundation.enum.ConductionWallGeometry.Planar  area=250 cm^2  thickness=30 cm  d_in=0.05 m  d_out=0.1 m  L=1 m  th_cond_min=10 W/(K*m)  th_cond=360 W/(m*K)  th_cond_TLU=[413, 401, 392, 383, 371, 357, 342] W/(K*m)  temp_TLU=[200, 273, 400, 600, 800, 1000, 1200] K  T_specify=off  T_priority=None  T=0 K  T_nominal_specify=off  T_nominal_value=1  T_nominal_unit=K  Q_specify=off  Q_priority=None  Q=0 W  Q_nominal_specify=off  Q_nominal_value=1  Q_nominal_unit=W
  WindingA-Iron Conductance1 : fl_lib/Thermal/Thermal Elements/Conductive Heat Transfer  Commented=on  thermal_type=foundation.enum.ConstantVariableTabulated.Constant  wall_geometry=foundation.enum.ConductionWallGeometry.Planar  area=250 cm^2  thickness=30 cm  d_in=0.05 m  d_out=0.1 m  L=1 m  th_cond_min=10 W/(K*m)  th_cond=360 W/(m*K)  th_cond_TLU=[413, 401, 392, 383, 371, 357, 342] W/(K*m)  temp_TLU=[200, 273, 400, 600, 800, 1000, 1200] K  T_specify=off  T_priority=None  T=0 K  T_nominal_specify=off  T_nominal_value=1  T_nominal_unit=K  Q_specify=off  Q_priority=None  Q=0 W  Q_nominal_specify=off  Q_nominal_value=1  Q_nominal_unit=W
  WindingB Thermal Mass : fl_lib/Thermal/Thermal Elements/Thermal Mass  Commented=on  mass_type=foundation.enum.constant_variable.constant  mass=6.3 kg  sp_heat=385 J/kg/K  mass_min=1e-6 kg  num_ports=foundation.enum.numPorts2.one  m_specify=off  m_priority=High  m=1 kg  m_nominal_specify=off  m_nominal_value=1  m_nominal_unit=kg  T_specify=off  T_priority=High  T=300 K  T_nominal_specify=off  T_nominal_value=1  T_nominal_unit=K  Q_specify=off  Q_priority=None  Q=0 W  Q_nominal_specify=off  Q_nominal_value=1  Q_nominal_unit=W
  WindingB-Iron Conductance : fl_lib/Thermal/Thermal Elements/Conductive Heat Transfer  Commented=on  thermal_type=foundation.enum.ConstantVariableTabulated.Constant  wall_geometry=foundation.enum.ConductionWallGeometry.Planar  area=250 cm^2  thickness=30 cm  d_in=0.05 m  d_out=0.1 m  L=1 m  th_cond_min=10 W/(K*m)  th_cond=360 W/(m*K)  th_cond_TLU=[413, 401, 392, 383, 371, 357, 342] W/(K*m)  temp_TLU=[200, 273, 400, 600, 800, 1000, 1200] K  T_specify=off  T_priority=None  T=0 K  T_nominal_specify=off  T_nominal_value=1  T_nominal_unit=K  Q_specify=off  Q_priority=None  Q=0 W  Q_nominal_specify=off  Q_nominal_value=1  Q_nominal_unit=W
  WindingB-Iron Conductance1 : fl_lib/Thermal/Thermal Elements/Conductive Heat Transfer  Commented=on  thermal_type=foundation.enum.ConstantVariableTabulated.Constant  wall_geometry=foundation.enum.ConductionWallGeometry.Planar  area=250 cm^2  thickness=30 cm  d_in=0.05 m  d_out=0.1 m  L=1 m  th_cond_min=10 W/(K*m)  th_cond=360 W/(m*K)  th_cond_TLU=[413, 401, 392, 383, 371, 357, 342] W/(K*m)  temp_TLU=[200, 273, 400, 600, 800, 1000, 1200] K  T_specify=off  T_priority=None  T=0 K  T_nominal_specify=off  T_nominal_value=1  T_nominal_unit=K  Q_specify=off  Q_priority=None  Q=0 W  Q_nominal_specify=off  Q_nominal_value=1  Q_nominal_unit=W
  WindingC Thermal Mass : fl_lib/Thermal/Thermal Elements/Thermal Mass  Commented=on  mass_type=foundation.enum.constant_variable.constant  mass=6.3 kg  sp_heat=385 J/kg/K  mass_min=1e-6 kg  num_ports=foundation.enum.numPorts2.one  m_specify=off  m_priority=High  m=1 kg  m_nominal_specify=off  m_nominal_value=1  m_nominal_unit=kg  T_specify=off  T_priority=High  T=300 K  T_nominal_specify=off  T_nominal_value=1  T_nominal_unit=K  Q_specify=off  Q_priority=None  Q=0 W  Q_nominal_specify=off  Q_nominal_value=1  Q_nominal_unit=W
  WindingC-Iron Conductance : fl_lib/Thermal/Thermal Elements/Conductive Heat Transfer  Commented=on  thermal_type=foundation.enum.ConstantVariableTabulated.Constant  wall_geometry=foundation.enum.ConductionWallGeometry.Planar  area=250 cm^2  thickness=30 cm  d_in=0.05 m  d_out=0.1 m  L=1 m  th_cond_min=10 W/(K*m)  th_cond=360 W/(m*K)  th_cond_TLU=[413, 401, 392, 383, 371, 357, 342] W/(K*m)  temp_TLU=[200, 273, 400, 600, 800, 1000, 1200] K  T_specify=off  T_priority=None  T=0 K  T_nominal_specify=off  T_nominal_value=1  T_nominal_unit=K  Q_specify=off  Q_priority=None  Q=0 W  Q_nominal_specify=off  Q_nominal_value=1  Q_nominal_unit=W
  WindingC-Iron Conductance1 : fl_lib/Thermal/Thermal Elements/Conductive Heat Transfer  Commented=on  thermal_type=foundation.enum.ConstantVariableTabulated.Constant  wall_geometry=foundation.enum.ConductionWallGeometry.Planar  area=250 cm^2  thickness=30 cm  d_in=0.05 m  d_out=0.1 m  L=1 m  th_cond_min=10 W/(K*m)  th_cond=360 W/(m*K)  th_cond_TLU=[413, 401, 392, 383, 371, 357, 342] W/(K*m)  temp_TLU=[200, 273, 400, 600, 800, 1000, 1200] K  T_specify=off  T_priority=None  T=0 K  T_nominal_specify=off  T_nominal_value=1  T_nominal_unit=K  Q_specify=off  Q_priority=None  Q=0 W  Q_nominal_specify=off  Q_nominal_value=1  Q_nominal_unit=W
  Conn1 : PMIOPort  Side=Right
  wires:
  Demux1/1 -> Square3/1
  Gain2/1 -> Mux4/3, Simulink-PS Converter2/1  "C winding"
  Square1/1 -> Gain1/1
  Mux4/1 -> Joule loss (J)/1
  Demux1/3 -> Square5/1
  Demux/3 -> Square2/1
  Square4/1 -> Gain4/1
  Square/1 -> Gain/1
  Gain3/1 -> Mux5/1, Simulink-PS Converter3/1  "A winding"
  Demux/1 -> Square/1
  Square3/1 -> Gain3/1
  Gain/1 -> Mux4/1, Simulink-PS Converter/1  "A winding"
  Gain5/1 -> Terminator2/1, Mux5/3  "C winding"
  Square5/1 -> Gain5/1
  Demux/2 -> Square1/1
  Gain4/1 -> Terminator1/1, Mux5/2  "B winding"
  Mux5/1 -> Joule loss (J)1/1
  Square2/1 -> Gain2/1
  Gain1/1 -> Simulink-PS Converter1/1, Mux4/2  "B winding"
  Demux1/2 -> Square4/1
  From4/1 -> Demux/1
  From10/1 -> Demux1/1
  connections:
  ThRef5/LConn1 -- Controlled Heat Flow Rate Source3/RConn2
  Controlled Heat Flow Rate Source/LConn1 -- Sensing Temperature WiA/LConn1 -- Thermal Resistance/LConn1 -- WindingA Thermal Mass/LConn1
  Sensing Temperature WiA3/LConn1 -- Temperature Source1/LConn1 -- Case-Atmosphere Convection1/RConn1
  WindingC Thermal Mass/LConn1 -- Thermal Resistance2/LConn1 -- Sensing Temperature WiC/LConn1 -- Controlled Heat Flow Rate Source2/LConn1
  Iron Stack-Case Conductance1/RConn1 -- Case-Atmosphere Convection1/LConn1 -- Motor Case Thermal Mass1/LConn1
  ThRef/LConn1 -- Temperature Source/RConn2
  WindingB Thermal Mass/LConn1 -- Thermal Resistance1/LConn1 -- Sensing Temperature WiB/LConn1 -- Controlled Heat Flow Rate Source1/LConn1
  ThRef1/LConn1 -- Temperature Source1/RConn2
  Controlled Heat Flow Rate Source3/RConn1 -- Simulink-PS Converter3/RConn1
  Iron Stack-Case Conductance/LConn1 -- Stator Iron Thermal Mass/LConn1
  Sensing Temperature WiA2/LConn1 -- Solver Configuration5/RConn1 -- WindingA-Iron Conductance1/LConn1 -- Controlled Heat Flow Rate Source3/LConn1 -- WindingA Thermal Mass1/LConn1
  Motor Case Thermal Mass/LConn1 -- Case-Atmosphere Convection/LConn1 -- Iron Stack-Case Conductance/RConn1
  ThRef2/LConn1 -- Controlled Heat Flow Rate Source/RConn2
  Solver Configuration4/RConn1 -- Thermal Resistance2/RConn1
  Controlled Heat Flow Rate Source2/RConn1 -- Simulink-PS Converter2/RConn1
  Ambient Temperature1/RConn1 -- Temperature Source1/RConn1
  Controlled Heat Flow Rate Source1/RConn1 -- Simulink-PS Converter1/RConn1
  ThRef3/LConn1 -- Controlled Heat Flow Rate Source1/RConn2
  Thermal Resistance1/RConn1 -- Solver Configuration3/RConn1
  Sensing Temperature WiA1/LConn1 -- Thermal Resistance/RConn1 -- Solver Configuration2/RConn1 -- Temperature Source/LConn1
  Ambient Temperature/RConn1 -- Temperature Source/RConn1
  ThRef4/LConn1 -- Controlled Heat Flow Rate Source2/RConn2
  Controlled Heat Flow Rate Source/RConn1 -- Simulink-PS Converter/RConn1
  Iron Stack-Case Conductance1/LConn1 -- WindingA-Iron Conductance1/RConn1 -- Stator Iron Thermal Mass1/LConn1
  Case-Atmosphere Convection/RConn1 -- Conn1/RConn1

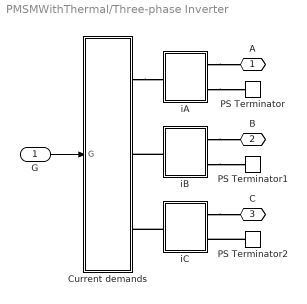
== system PMSMWithThermal/Three-phase Inverter ==
  G : Inport
  Current demands : Subsystem
  PS Terminator : fl_lib/Physical Signals/Sinks/PS Terminator
  PS Terminator1 : fl_lib/Physical Signals/Sinks/PS Terminator
  PS Terminator2 : fl_lib/Physical Signals/Sinks/PS Terminator
  iA : Subsystem
  iB : Subsystem
  iC : Subsystem
  A : PMIOPort  Tag=PMCPort  Side=Right
  B : PMIOPort  Tag=PMCPort  Port=2  Side=Right
  C : PMIOPort  Tag=PMCPort  Port=3  Side=Right
  wires:
  G/1 -> Current demands/1(G)
  connections:
  iA/RConn1 -- A/RConn1
  Current demands/RConn1 -- iA/LConn1
  iB/LConn1 -- Current demands/RConn2
  iC/LConn1 -- Current demands/RConn3
  iB/RConn1 -- B/RConn1
  iC/RConn1 -- C/RConn1
  iA/RConn2 -- PS Terminator/LConn1
  PS Terminator2/LConn1 -- iC/RConn2
  iB/RConn2 -- PS Terminator1/LConn1

== system PMSMWithThermal/cogging_torque ==
  th_mech : Inport
  Gain : Gain  Gain=N
  Gain1 : Gain  Gain=10^3
  MATLAB Function : MATLAB Function  TreatAsAtomicUnit=on
  Mod : Math  Operator=mod  SignedPower=on
  Pi : Constant  Value=2*pi  OutDataTypeStr=Inherit: Inherit via back propagation
  T : Outport
  wires:
  Gain/1 -> Mod/1
  th_mech/1 -> Gain/1
  Pi/1 -> Mod/2
  Mod/1 -> MATLAB Function/1(theta_e)
  MATLAB Function/1(T) -> Gain1/1
  Gain1/1 -> T/1

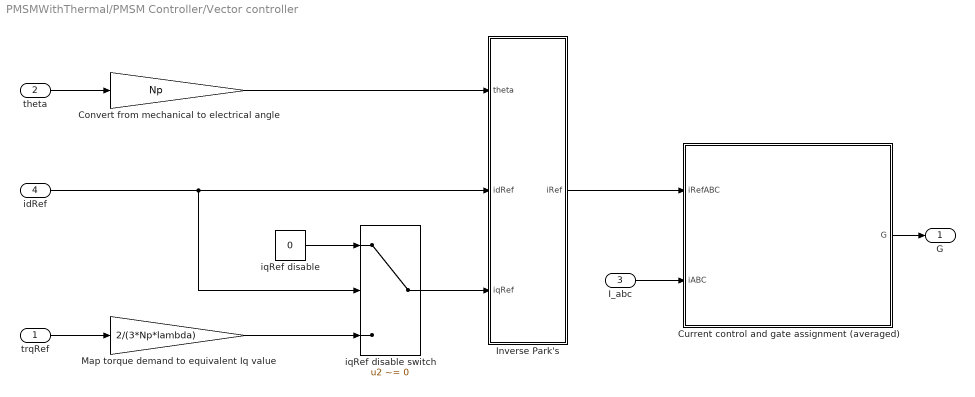
== system PMSMWithThermal/PMSM Controller/Vector controller ==
  trqRef : Inport
  theta : Inport  Port=2
  I_abc : Inport  Port=3
  idRef : Inport  Port=4
  Convert from mechanical to electrical angle : Gain  Gain=Np  SaturateOnIntegerOverflow=on  OutDataTypeStr=Inherit: Same as input  ParamDataTypeStr=Inherit: Same as input
  Current control and gate assignment (averaged) : Subsystem  VariantControl=Variant1
  Inverse Park's : Subsystem
  Map torque demand to equivalent Iq value : Gain  Gain=2/(3*Np*lambda)  SaturateOnIntegerOverflow=on  OutDataTypeStr=Inherit: Same as input  ParamDataTypeStr=Inherit: Same as input
  iqRef disable : Constant  Value=0
  iqRef disable switch : Switch  Criteria=u2 ~= 0  SaturateOnIntegerOverflow=off  InputSameDT=off
  G : Outport  VectorParamsAs1DForOutWhenUnconnected=off
  wires:
  Current control and gate assignment (averaged)/1(G) -> G/1
  I_abc/1 -> Current control and gate assignment (averaged)/2(iABC)
  Inverse Park's/1(iRef) -> Current control and gate assignment (averaged)/1(iRefABC)
  trqRef/1 -> Map torque demand to equivalent Iq value/1
  theta/1 -> Convert from mechanical to electrical angle/1
  Convert from mechanical to electrical angle/1 -> Inverse Park's/1(theta)
  iqRef disable switch/1 -> Inverse Park's/3(iqRef)
  idRef/1 -> Inverse Park's/2(idRef), iqRef disable switch/2
  Map torque demand to equivalent Iq value/1 -> iqRef disable switch/3
  iqRef disable/1 -> iqRef disable switch/1

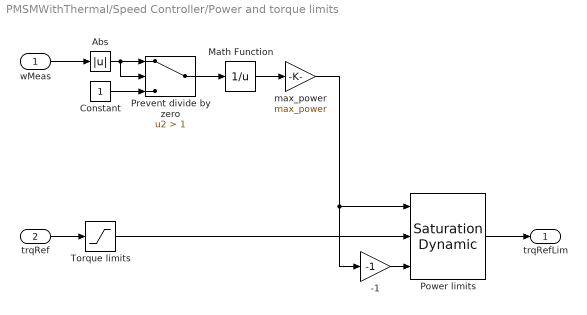
== system PMSMWithThermal/Speed Controller/Power and torque limits ==
  wMeas : Inport
  trqRef : Inport  Port=2
  -1 : Gain  Gain=-1
  Abs : Abs  SaturateOnIntegerOverflow=off
  Constant : Constant  SampleTime=dt_speed_control
  Math Function : Math  Operator=reciprocal  SignedPower=on
  Power limits : simulink/Discontinuities/Saturation Dynamic  OutMin=[]  OutMax=[]  OutDataTypeStr=Inherit: Same as second input  OutDataType=fixdt(1, 16)  OutScaling=2^-10  DoSatur=off
  Prevent divide by zero : Switch  Criteria=u2 > Threshold  Threshold=1  SaturateOnIntegerOverflow=off  InputSameDT=off
  Torque limits : Saturate  UpperLimit=max_torque  LowerLimit=-max_torque
  max_power : Gain  Gain=max_power
  trqRefLim : Outport  VectorParamsAs1DForOutWhenUnconnected=off
  wires:
  wMeas/1 -> Abs/1
  -1/1 -> Power limits/3
  Constant/1 -> Prevent divide by zero/3
  Prevent divide by zero/1 -> Math Function/1
  max_power/1 -> -1/1, Power limits/1
  Math Function/1 -> max_power/1
  Torque limits/1 -> Power limits/2
  Abs/1 -> Prevent divide by zero/1, Prevent divide by zero/2
  trqRef/1 -> Torque limits/1
  Power limits/1 -> trqRefLim/1

== system PMSMWithThermal/Speed Controller/Speed controller ==
  wMeas : Inport
  wRef : Inport  Port=2
  Speed controller : Subsystem  mask(P+I motor speed controller){Kp=300, Ki=300, trqMax=max_torque, ts=dt_speed_control}
      mask prompts: Kp "Proportional gain (Nm/(rad/s))"; Ki "Integral gain (Nm/rad)"; trqMax "Maximum torque demand"; ts "Sample time"
      mask help: Inputs wRef and wMeas are the demanded rotor speed and measured rotor speed in rad/s. The controller output is a torque demand in Nm.
  trqRef : Outport  VectorParamsAs1DForOutWhenUnconnected=off
  tag scope: wDemand=global
  wires:
  wRef/1 -> Speed controller/1(wRef), [wDemand]
  Speed controller/1(trqRef) -> trqRef/1
  wMeas/1 -> Speed controller/2(wMeas)

== system PMSMWithThermal/Thermal network model/Sensing Temperature WiA ==
  PS-Simulink Converter : nesl_utility/PS-Simulink Converter  PhysicalDomain=network_engine_domain  SubClassName=ps_output  LeftPortType=input  RightPortType=output  PseudoPeriodic=off  Frequencies=[]  VectorFormat=1-D array  Unit=degC  AffineConversion=on
  Temperature Sensor : fl_lib/Thermal/Thermal Sensors/Temperature Sensor  temperature_measure=foundation.enum.MeasurementReference.difference
  ThRef : fl_lib/Thermal/Thermal Elements/Thermal Reference
  H : PMIOPort  Side=Left
  tag scope: TA=global
  wires:
  PS-Simulink Converter/1 -> [TA]
  connections:
  H/RConn1 -- Temperature Sensor/LConn1
  ThRef/LConn1 -- Temperature Sensor/RConn1
  Temperature Sensor/RConn2 -- PS-Simulink Converter/LConn1

== system PMSMWithThermal/Thermal network model/Sensing Temperature WiA1 ==
  PS-Simulink Converter : nesl_utility/PS-Simulink Converter  PhysicalDomain=network_engine_domain  SubClassName=ps_output  LeftPortType=input  RightPortType=output  PseudoPeriodic=off  Frequencies=[]  VectorFormat=1-D array  Unit=degC  AffineConversion=on
  Temperature Sensor : fl_lib/Thermal/Thermal Sensors/Temperature Sensor  temperature_measure=foundation.enum.MeasurementReference.difference
  ThRef : fl_lib/Thermal/Thermal Elements/Thermal Reference
  H : PMIOPort  Side=Left
  tag scope: Ta=global
  wires:
  PS-Simulink Converter/1 -> [Ta]
  connections:
  H/RConn1 -- Temperature Sensor/LConn1
  ThRef/LConn1 -- Temperature Sensor/RConn1
  Temperature Sensor/RConn2 -- PS-Simulink Converter/LConn1

== system PMSMWithThermal/Thermal network model/Sensing Temperature WiA2 ==
  PS-Simulink Converter : nesl_utility/PS-Simulink Converter  PhysicalDomain=network_engine_domain  SubClassName=ps_output  LeftPortType=input  RightPortType=output  PseudoPeriodic=off  Frequencies=[]  VectorFormat=1-D array  Unit=degC  AffineConversion=on
  Temperature Sensor : fl_lib/Thermal/Thermal Sensors/Temperature Sensor  temperature_measure=foundation.enum.MeasurementReference.difference
  ThRef : fl_lib/Thermal/Thermal Elements/Thermal Reference
  H : PMIOPort  Side=Left
  tag scope: TA=global
  wires:
  PS-Simulink Converter/1 -> [TA]
  connections:
  H/RConn1 -- Temperature Sensor/LConn1
  ThRef/LConn1 -- Temperature Sensor/RConn1
  Temperature Sensor/RConn2 -- PS-Simulink Converter/LConn1

== system PMSMWithThermal/Thermal network model/Sensing Temperature WiA3 ==
  PS-Simulink Converter : nesl_utility/PS-Simulink Converter  PhysicalDomain=network_engine_domain  SubClassName=ps_output  LeftPortType=input  RightPortType=output  PseudoPeriodic=off  Frequencies=[]  VectorFormat=1-D array  Unit=degC  AffineConversion=on
  Temperature Sensor : fl_lib/Thermal/Thermal Sensors/Temperature Sensor  temperature_measure=foundation.enum.MeasurementReference.difference
  ThRef : fl_lib/Thermal/Thermal Elements/Thermal Reference
  H : PMIOPort  Side=Left
  tag scope: Ta=global
  wires:
  PS-Simulink Converter/1 -> [Ta]
  connections:
  H/RConn1 -- Temperature Sensor/LConn1
  ThRef/LConn1 -- Temperature Sensor/RConn1
  Temperature Sensor/RConn2 -- PS-Simulink Converter/LConn1

== system PMSMWithThermal/Thermal network model/Sensing Temperature WiB ==
  PS-Simulink Converter : nesl_utility/PS-Simulink Converter  PhysicalDomain=network_engine_domain  SubClassName=ps_output  LeftPortType=input  RightPortType=output  PseudoPeriodic=off  Frequencies=[]  VectorFormat=1-D array  Unit=degC  AffineConversion=on
  Temperature Sensor : fl_lib/Thermal/Thermal Sensors/Temperature Sensor  temperature_measure=foundation.enum.MeasurementReference.difference
  ThRef : fl_lib/Thermal/Thermal Elements/Thermal Reference
  H : PMIOPort  Side=Left
  tag scope: TB=global
  wires:
  PS-Simulink Converter/1 -> [TB]
  connections:
  Temperature Sensor/RConn2 -- PS-Simulink Converter/LConn1
  ThRef/LConn1 -- Temperature Sensor/RConn1
  H/RConn1 -- Temperature Sensor/LConn1

== system PMSMWithThermal/Thermal network model/Sensing Temperature WiC ==
  PS-Simulink Converter : nesl_utility/PS-Simulink Converter  PhysicalDomain=network_engine_domain  SubClassName=ps_output  LeftPortType=input  RightPortType=output  PseudoPeriodic=off  Frequencies=[]  VectorFormat=1-D array  Unit=degC  AffineConversion=on
  Temperature Sensor : fl_lib/Thermal/Thermal Sensors/Temperature Sensor  temperature_measure=foundation.enum.MeasurementReference.difference
  ThRef : fl_lib/Thermal/Thermal Elements/Thermal Reference
  H : PMIOPort  Side=Left
  tag scope: TC=global
  wires:
  PS-Simulink Converter/1 -> [TC]
  connections:
  H/RConn1 -- Temperature Sensor/LConn1
  ThRef/LConn1 -- Temperature Sensor/RConn1
  Temperature Sensor/RConn2 -- PS-Simulink Converter/LConn1
